simulink model "sm_car_test_ggv_new"  (R2026a)
settings: Solver=ode23t  StopTime=300  MaxStep=0.4  AbsTol=1e-3  EnableMultiTasking=on
PreLoadFcn:
  | % PreLoadFcn Removed for GGV Sweep
PostLoadFcn:
  | % PostLoadFcn Removed for GGV Sweep
InitFcn:
  | sm_car_config_camera;
  | Vehicle = sm_car_vehcfg_checkConfig(Vehicle);
  | sm_car_check_tire_model(bdroot);
StartFcn:
  | tic;
StopFcn:
  | Elapsed_Sim_Time = toc;
  | % disp(['Elapsed Sim Time = ' num2str(Elapsed_Sim_Time)]);
values from neighbouring files (symbols this model uses):
  accel_ramp_rate = 0.1    [sm_car_sweep_ggv_pts.m]
undefined symbols (not defined in the file or in its folder): acc_theta, Axle1D, AxleIn, Camera, Control, drag_frc, Driver, Init, lift_frc, Maneuver, Pedal, Scene, ShaftL1, ShaftL2, ShaftR1, ShaftR2, Visual, X, xy_data_car_side, Y, Z
libraries: sm_lib x270, fl_lib x171, nesl_utility x137, simulink x56, sdl_lib x14, simulink_extras x11, SimscapeFluids_lib x7, Scene_Utilities x6, dspsigops x4, Damper_Element x4, Tire_1x2x x4, ee_lib x3
(part 5 of 20)

== system sm_car_test_ggv_new/World/Scene ==
  CRG Dej : sm_car_scene_crg_dej/CRG Dej  VariantControl=CRG_Dej  geometry=Scene.CRG_Dej.Geometry
  CRG Dej F : sm_car_scene_crg_dej_f/CRG Dej F  VariantControl=CRG_Dej_F  geometry=Scene.CRG_Dej_F.Geometry
  CRG Dej Wide : sm_car_scene_crg_dej_wide/CRG Dej Wide  VariantControl=CRG_Dej_Wide  geometry=Scene.CRG_Dej_Wide.Geometry
  CRG Dej Wide F : sm_car_scene_crg_dej_wide_f/CRG Dej Wide F  VariantControl=CRG_Dej_Wide_F  geometry=Scene.CRG_Dej_Wide_F.Geometry
  CRG Germania : sm_car_scene_crg_germania/CRG Germania  VariantControl=CRG_Germania  geometry=Scene.CRG_Germania.Geometry
  CRG Germania F : sm_car_scene_crg_germania_f/CRG Germania F  VariantControl=CRG_Germania_F  geometry=Scene.CRG_Germania_F.Geometry
  CRG Hockenheim : Subsystem  VariantControl=CRG_Hockenheim  mask{geometry=Scene.CRG_Hockenheim.Geometry}
      mask prompts: geometry "Geometry (structure)"
  CRG Hockenheim F : Subsystem  VariantControl=CRG_Hockenheim_F  mask{geometry=Scene.CRG_Hockenheim_F.Geometry}
      mask prompts: geometry "Geometry (structure)"
  CRG Teste : sm_car_scene_crg_teste/CRG Teste  VariantControl=CRG _Teste  geometry=Scene.CRG_Teste.Geometry
  CRG Teste F : sm_car_scene_crg_teste_f/CRG Teste F  VariantControl=CRG_Teste_F  geometry=Scene.CRG_Teste_F.Geometry
  Double Lane Change : Subsystem  VariantControl=Double_Lane_Change  mask{road=Scene.Double_Lane_Change.Road, dashes=Scene.Double_Lane_Change.Dashes, cones=Scene.Double_Lane_Change.Cones}
      mask prompts: road "Road (structure)"; dashes "Dashes (structure)"; cones "Cones (structure)"
  Double Lane Change ISO3888 : Subsystem  VariantControl=Double_Lane_Change_ISO3888  mask{road=Scene.Double_Lane_Change_ISO3888.Road, dashes=Scene.Double_Lane_Change_ISO3888.Dashes, cones=Scene.Double_Lane_Change_ISO3888.Cones}
      mask prompts: road "Road (structure)"; dashes "Dashes (structure)"; cones "Cones (structure)"
  Plane Grid : Subsystem  VariantControl=Plane_Grid  mask{plane=Scene.Plane_Grid.Plane, grid=Scene.Plane_Grid.Grid}
      mask prompts: plane "Ground Plane (structure)"; grid "Grid (structure)"
  Skidpad : Subsystem  VariantControl=Skidpad  mask{circ_in=Scene.Skidpad.Circle_Inner, circ_out=Scene.Skidpad.Circle_Outer, plane=Scene.Skidpad.Plane}
      mask prompts: circ_in "Circle Inner (structure)"; circ_out "Circle Outer (structure)"; plane "Plane (structure)"
  W : PMIOPort  Side=Left
  Obs : Outport  VectorParamsAs1DForOutWhenUnconnected=off

== system sm_car_test_ggv_new/Camera Frames/Dolly Camera/Off ==
  W : PMIOPort  Side=Left
  R : PMIOPort  Port=2  Side=Right
  connections:
  R/RConn1 -- W/RConn1

== system sm_car_test_ggv_new/Controller/Default/Brake Control ==
  "rBrakePedal " : Inport
  "VehBus " : Inport  Port=2
  Pedal : Subsystem  VariantControl=Pedal
  " Brakes" : Outport  VectorParamsAs1DForOutWhenUnconnected=off

== system sm_car_test_ggv_new/Controller/Default/Driveline Control ==
  Bus Creator : BusCreator  Inputs=1
  Constant : Constant  Value=0
  Driveline : Outport  VectorParamsAs1DForOutWhenUnconnected=off
  wires:
  Bus Creator/1 -> Driveline/1  "Driveline"
  Constant/1 -> Bus Creator/1  "placeholder"

== system sm_car_test_ggv_new/Controller/Default/Power Control ==
  note: For 4 Motor Powertrain only
  note: For 2 Motor Powertrain only
  rAccelPedal : Inport
  VehBus : Inport  Port=2
  StatesEst : Inport  Port=3
  Bus Creator : BusCreator  Inputs=7
  Constant : Constant  Value=trq_ratio_front
  Constant1 : Constant  Value=0
  Constant2 : Constant
  Gain : Gain  Gain=max(Vehicle.Powertrain.Power.Motor.TorqueSpd.trq.Value)
  Gain1 : Gain
  Gain2 : Gain
  Gain3 : Gain  Gain=0.5
  Gain4 : Gain  Gain=0.5
  Product : Product
  Product1 : Product
  Rate Limiter : RateLimiter  RisingSlewLimit=trq_rate_up  FallingSlewLimit=trq_rate_down  SampleTimeMode=inherited
  Terminator : Terminator
  Terminator1 : Terminator
  Power : Outport  VectorParamsAs1DForOutWhenUnconnected=off
  wires:
  Bus Creator/1 -> Power/1  "Power"
  Product1/1 -> Gain2/1, Gain1/1, Bus Creator/4  "MMotorA2Demand"
  Gain/1 -> Rate Limiter/1
  Product/1 -> Gain4/1, Gain3/1, Bus Creator/1  "MMotorA1Demand"
  rAccelPedal/1 -> Gain/1
  VehBus/1 -> Terminator/1
  Constant1/1 -> Bus Creator/7  "MRegenBrakeLimit"
  Rate Limiter/1 -> Product1/1, Product/2
  Constant/1 -> Product/1
  Constant2/1 -> Product1/2
  Gain1/1 -> Bus Creator/5  "MMotorL2Demand"
  Gain2/1 -> Bus Creator/6  "MMotorR2Demand"
  Gain3/1 -> Bus Creator/2  "MMotorL1Demand"
  Gain4/1 -> Bus Creator/3  "MMotorR1Demand"
  StatesEst/1 -> Terminator1/1

== system sm_car_test_ggv_new/Controller/Default/Spring Damper ==
  Bus Creator : BusCreator  Inputs=4
  Bus Creator1 : BusCreator  Inputs=4
  Constant : Constant  Value=[0 0 0 0]
  Constant1 : Constant  Value=[0 0 0 0]
  Demux : Demux
  Demux1 : Demux
  Damper : Outport  VectorParamsAs1DForOutWhenUnconnected=off
  Spring : Outport  Port=2  VectorParamsAs1DForOutWhenUnconnected=off
  wires:
  Constant/1 -> Demux/1
  Demux/3 -> Bus Creator/3  "L2"
  Demux/4 -> Bus Creator/4  "R2"
  Demux/1 -> Bus Creator/1  "L1"
  Demux/2 -> Bus Creator/2  "R1"
  Demux1/2 -> Bus Creator1/2  "R1"
  Demux1/1 -> Bus Creator1/1  "L1"
  Demux1/4 -> Bus Creator1/4  "R2"
  Demux1/3 -> Bus Creator1/3  "L2"
  Constant1/1 -> Demux1/1
  Bus Creator1/1 -> Damper/1  "Damper"
  Bus Creator/1 -> Spring/1  "Spring"

== system sm_car_test_ggv_new/Controller/Default/State Estimation ==
  aSteerWheel : Inport
  VehBus : Inport  Port=2
  Bus Creator : BusCreator  Inputs=6
  Bus Selector : BusSelector  OutputSignals=Chassis.Body.CG.vx,World.vx,World.vy,World.vz,Chassis.Body.CG.aYaw,Chassis.Body.CG.nYaw,Chassis.Body.CG.gx,Chassis.Body.CG.gy,Chassis.SuspA1.LinkageL.Upright.Upright.w,Chassis.SuspA1.LinkageR.Upright.Upright.w,Chassis.SuspA2.LinkageL.Upright.Upright.w,Chassis.SuspA2.LinkageR.Upright.Upright.w
  Compare To Constant : simulink/Logic and Bit Operations/Compare To Constant  relop=>=  const=0.4  OutDataTypeStr=boolean
  Data Type Conversion : DataTypeConversion  OutDataTypeStr=double  SaturateOnIntegerOverflow=off  RndMeth=Floor
  Demux : Demux  Outputs=6
  Rate Transition1 : RateTransition  Deterministic=off  OutPortSampleTime=0.003
  Rate Transition2 : RateTransition  Deterministic=off  OutPortSampleTime=0.003
  Rate Transition3 : RateTransition  Deterministic=off  OutPortSampleTime=0.003
  Sensor Noise Simulation : Subsystem
  Subsystem : Subsystem
  StateEst : Outport
  Out Bus Element : Outport  Port=2  PortName=Meas  Element=Meas
  Out Bus Element1 : Outport  Port=2  PortName=Meas  Element=Input
  Out Bus Element2 : Outport  Port=2  PortName=Meas  Element=State
  wires:
  VehBus/1 -> Bus Selector/1
  Bus Selector/2 -> Sensor Noise Simulation/1(<vx>)  "<vx>"
  Bus Selector/3 -> Sensor Noise Simulation/2(<vy>)  "<vy>"
  Bus Selector/5 -> Sensor Noise Simulation/4(<aYaw>)  "<aYaw>"
  Bus Selector/6 -> Sensor Noise Simulation/5(<nYaw>)  "<nYaw>"
  Bus Selector/7 -> Sensor Noise Simulation/6(<gx>)  "<gx>"
  Bus Selector/8 -> Sensor Noise Simulation/7(<gy>)  "<gy>"
  Bus Selector/9 -> Sensor Noise Simulation/8(<w_fl>)  "<w>"
  Bus Selector/10 -> Sensor Noise Simulation/9(<w_fr>)  "<w>"
  Bus Selector/11 -> Sensor Noise Simulation/10(<w_rl>)  "<w>"
  Bus Selector/12 -> Sensor Noise Simulation/11(<w_rr>)  "<w>"
  aSteerWheel/1 -> Sensor Noise Simulation/12(delta)  "delta"
  Sensor Noise Simulation/2(Meas) -> Out Bus Element/1, Rate Transition2/1  "Measument"
  Sensor Noise Simulation/1(Inputs) -> Out Bus Element1/1, Rate Transition1/1  "Input"
  Bus Selector/4 -> Sensor Noise Simulation/3(<vz>)  "<vz>"
  Data Type Conversion/1 -> Demux/1
  Bus Creator/1 -> Out Bus Element2/1, StateEst/1  "UKF"
  Demux/1 -> Bus Creator/1  "v_x"
  Demux/2 -> Bus Creator/2  "v_y"
  Demux/3 -> Bus Creator/3  "phi"
  Demux/4 -> Bus Creator/4  "phi_dot"
  Demux/5 -> Bus Creator/5  "a_x"
  Demux/6 -> Bus Creator/6  "a_y"
  Compare To Constant/1 -> Rate Transition3/1
  Rate Transition3/1 -> Subsystem/Enable
  Rate Transition1/1 -> Subsystem/1(StateTransitionFcnInputs)
  Rate Transition2/1 -> Subsystem/2(y1)
  Subsystem/1(xhat) -> Data Type Conversion/1
  Bus Selector/1 -> Compare To Constant/1  "<vx>"

== system sm_car_test_ggv_new/Controller/Default/Susp ==
  aSteerWheel : Inport
  vx : Inport  Port=2
  1-D Lookup Table : Lookup_n-D  NumberOfTableDimensions=1  BreakpointsForDimension1=Steer.Gain.vVehicle.Value  Table=Steer.Gain.n.Value  InterpMethod=Linear Lagrange  InternalRulePriority=Speed  RndMeth=Simplest
  Bus Creator{1..4} (4 alike) : BusCreator  Inputs=1
  Gain : Gain  Gain=3.6
  Product : Product
  Saturation : Saturate  UpperLimit=Steer.Limits.aUpper.Value  LowerLimit=Steer.Limits.aLower.Value  LinearizeAsGain=off  ZeroCross=off
  Transfer Fcn (with initial states) : simulink_extras/Additional Linear/Transfer Fcn (with initial states)  N=[1]  D="[1/Steer.fActuatorCutoff.Value  1]"  X0=-1
  SuspA1 : Outport  VectorParamsAs1DForOutWhenUnconnected=off
  SuspA2 : Outport  Port=2  VectorParamsAs1DForOutWhenUnconnected=off
  wires:
  Bus Creator4/1 -> Bus Creator1/1  "Steer"
  Bus Creator2/1 -> Bus Creator3/1  "Steer"
  Bus Creator3/1 -> SuspA2/1  "SuspA2"
  Bus Creator1/1 -> SuspA1/1  "SuspA1"
  aSteerWheel/1 -> Product/1, Bus Creator4/1  "aSteerWheel"
  Saturation/1 -> Bus Creator2/1  "aSteerWheel"
  vx/1 -> Gain/1
  Transfer Fcn (with initial states)/1 -> Product/2
  Product/1 -> Saturation/1
  Gain/1 -> 1-D Lookup Table/1
  1-D Lookup Table/1 -> Transfer Fcn (with initial states)/1

== system sm_car_test_ggv_new/Controller/FeedF_Ctrl/Brake Control ==
  "rBrakePedal " : Inport
  "VehBus " : Inport  Port=2
  Pedal : Subsystem  VariantControl=Pedal
  " Brakes" : Outport  VectorParamsAs1DForOutWhenUnconnected=off

== system sm_car_test_ggv_new/Controller/FeedF_Ctrl/Driveline Control ==
  Bus Creator : BusCreator  Inputs=1
  Constant : Constant  Value=0
  Driveline : Outport  VectorParamsAs1DForOutWhenUnconnected=off
  wires:
  Constant/1 -> Bus Creator/1  "placeholder"
  Bus Creator/1 -> Driveline/1  "Driveline"

== system sm_car_test_ggv_new/Controller/FeedF_Ctrl/Power Control ==
  rAccelPedal : Inport
  VehBus : Inport  Port=2
  aSteerWheel : Inport  Port=3
  Bias : Bias  Bias=512  SaturateOnIntegerOverflow=off
  Bus Creator : BusCreator  Inputs=2
  Bus Selector : BusSelector  OutputSignals=Power.MotorL2.w,Power.MotorR2.w
  Gain : Gain  Gain=max(Control.MotorTrq)
  Gain1 : Gain  Gain=max(Control.MotorTrq)
  Gain3 : Gain  Gain=511/154
  Radians to Degrees : simulink_extras/Transformations/Radians to Degrees
  Subsystem Reference : Subsystem  ReferencedSubsystem=FeedForward  rwheel=Control.WheelRad  L=Control.Wheelbase  StrWhlRatio=Control.StrWheelRatio  Izz=Control.Izz  tr=Control.RearTrack  Gr=Control.GearRatio  MotorT=Control.MotorTrq  MotorW=Control.MotorW  Tf=0.005  Tmax=max(Control.MotorTrq)  Ku=Control.UndersteerGradient
  Power : Outport  VectorParamsAs1DForOutWhenUnconnected=off
  wires:
  Bias/1 -> Subsystem Reference/1
  Gain3/1 -> Bias/1
  Radians to Degrees/1 -> Gain3/1
  Gain1/1 -> Bus Creator/2  "MMotorR2Demand"
  Gain/1 -> Bus Creator/1  "MMotorL2Demand"
  Subsystem Reference/2 -> Gain1/1  "MMotorR2Demand"
  Subsystem Reference/1 -> Gain/1  "MMotorL2Demand"
  Bus Creator/1 -> Power/1
  rAccelPedal/1 -> Subsystem Reference/4  "Throttle[~]"
  aSteerWheel/1 -> Radians to Degrees/1  "Throttle[~]"
  VehBus/1 -> Bus Selector/1
  Bus Selector/1 -> Subsystem Reference/2  "<w>"
  Bus Selector/2 -> Subsystem Reference/3  "<w>"

== system sm_car_test_ggv_new/Controller/FeedF_Ctrl/Spring Damper ==
  Bus Creator : BusCreator  Inputs=4
  Bus Creator1 : BusCreator  Inputs=4
  Constant : Constant  Value=[0 0 0 0]
  Constant1 : Constant  Value=[0 0 0 0]
  Demux : Demux
  Demux1 : Demux
  Damper : Outport  VectorParamsAs1DForOutWhenUnconnected=off
  Spring : Outport  Port=2  VectorParamsAs1DForOutWhenUnconnected=off
  wires:
  Bus Creator/1 -> Spring/1  "Spring"
  Bus Creator1/1 -> Damper/1  "Damper"
  Constant1/1 -> Demux1/1
  Demux1/3 -> Bus Creator1/3  "L2"
  Demux1/4 -> Bus Creator1/4  "R2"
  Demux1/1 -> Bus Creator1/1  "L1"
  Demux1/2 -> Bus Creator1/2  "R1"
  Demux/2 -> Bus Creator/2  "R1"
  Demux/1 -> Bus Creator/1  "L1"
  Demux/4 -> Bus Creator/4  "R2"
  Demux/3 -> Bus Creator/3  "L2"
  Constant/1 -> Demux/1

== system sm_car_test_ggv_new/Controller/FeedF_Ctrl/Susp ==
  aSteerWheel : Inport
  vx : Inport  Port=2
  1-D Lookup Table : Lookup_n-D  NumberOfTableDimensions=1  BreakpointsForDimension1=Steer.Gain.vVehicle.Value  Table=Steer.Gain.n.Value  InterpMethod=Linear Lagrange  InternalRulePriority=Speed  RndMeth=Simplest
  Bus Creator{1..4} (4 alike) : BusCreator  Inputs=1
  Gain : Gain  Gain=3.6
  Product : Product
  Saturation : Saturate  UpperLimit=Steer.Limits.aUpper.Value  LowerLimit=Steer.Limits.aLower.Value  LinearizeAsGain=off  ZeroCross=off
  Transfer Fcn (with initial states) : simulink_extras/Additional Linear/Transfer Fcn (with initial states)  N=[1]  D="[1/Steer.fActuatorCutoff.Value  1]"  X0=-1
  SuspA1 : Outport  VectorParamsAs1DForOutWhenUnconnected=off
  SuspA2 : Outport  Port=2  VectorParamsAs1DForOutWhenUnconnected=off
  wires:
  1-D Lookup Table/1 -> Transfer Fcn (with initial states)/1
  Gain/1 -> 1-D Lookup Table/1
  Product/1 -> Saturation/1
  Transfer Fcn (with initial states)/1 -> Product/2
  vx/1 -> Gain/1
  Saturation/1 -> Bus Creator2/1  "aSteerWheel"
  aSteerWheel/1 -> Bus Creator4/1, Product/1  "aSteerWheel"
  Bus Creator1/1 -> SuspA1/1  "SuspA1"
  Bus Creator3/1 -> SuspA2/1  "SuspA2"
  Bus Creator2/1 -> Bus Creator3/1  "Steer"
  Bus Creator4/1 -> Bus Creator1/1  "Steer"

== system sm_car_test_ggv_new/Controller/NoIMU/Brake Control ==
  "rBrakePedal " : Inport
  "VehBus " : Inport  Port=2
  Pedal : Subsystem  VariantControl=Pedal
  " Brakes" : Outport  VectorParamsAs1DForOutWhenUnconnected=off

== system sm_car_test_ggv_new/Controller/NoIMU/Driveline Control ==
  Bus Creator : BusCreator  Inputs=1
  Constant : Constant  Value=0
  Driveline : Outport  VectorParamsAs1DForOutWhenUnconnected=off
  wires:
  Constant/1 -> Bus Creator/1  "placeholder"
  Bus Creator/1 -> Driveline/1  "Driveline"

== system sm_car_test_ggv_new/Controller/NoIMU/Power Control ==
  rAccelPedal : Inport
  VehBus : Inport  Port=2
  Add1 : Sum
  Bus Creator : BusCreator  Inputs=2
  Bus Creator2 : BusCreator  Inputs=2
  Bus Selector : BusSelector  OutputSignals=Power.Battery.v,Power.MotorL2.i,Power.MotorR2.i
  Constant : Constant
  Current-Torque : Subsystem
  Delay : Delay  DelayLength=1  InputProcessing=Columns as channels (frame based)
  Fuzzy Logic Controller : fuzblock/Fuzzy Logic  Controller  FIS=fis  OutputSampleNumber=101  DataType=double  UseLookupTable=off  NumBreakpoints=10  FuzzifiedInputs=off  RuleFiringStrengths=off  RuleOutputs=off  AggregatedOutputs=off  SimulateUsing=Interpreted execution  OutOfRangeInputValueMessage=warning  NoRuleFiredMessage=warning  EmptyOutputFuzzySetMessage=warning
  Product : Product
  Product1 : Product
  Product2 : Product  Inputs=3
  Saturation : Saturate  UpperLimit=1  LowerLimit=0
  Slip Control : Subsystem  Commented=on
  Subtract : Sum  Inputs=+-
  Sum : Sum  Inputs=|+-
  Tmax : Gain  Gain=1/Tmax/2
  max torque : Constant  Value=Tmax
  Power : Outport  VectorParamsAs1DForOutWhenUnconnected=off
  wires:
  VehBus/1 -> Slip Control/1(VehBus), Bus Selector/1
  Bus Creator/1 -> Power/1  "Power"
  rAccelPedal/1 -> Sum/1, Product2/1  "Throttle[~]"
  Bus Selector/1 -> Current-Torque/1(V)  "<v>"
  Bus Selector/2 -> Current-Torque/2(Il)  "<i>"
  Bus Selector/3 -> Current-Torque/3(Ir)  "<i>"
  Fuzzy Logic Controller/1 -> Add1/2
  Current-Torque/1(Out1) -> Tmax/1  "Treal[Nm]"
  Bus Creator2/1 -> ?
  Product2/1 -> Product/1, Product1/1  "MDemand[Nm]"
  Tmax/1 -> Saturation/1
  Saturation/1 -> Sum/2  "Treal[%]"
  max torque/1 -> Product2/3
  Add1/1 -> Product2/2
  Sum/1 -> Delay/1, Subtract/1, Bus Creator2/1
  Delay/1 -> Subtract/2
  Subtract/1 -> Bus Creator2/2
  Constant/1 -> Add1/1
  Product/1 -> Bus Creator/2  "MMotorR2Demand"
  Product1/1 -> Bus Creator/1  "MMotorL2Demand"
  Slip Control/1(Out1) -> Product1/2
  Slip Control/2(Out2) -> Product/2

== system sm_car_test_ggv_new/Controller/NoIMU/Spring Damper ==
  Bus Creator : BusCreator  Inputs=4
  Bus Creator1 : BusCreator  Inputs=4
  Constant : Constant  Value=[0 0 0 0]
  Constant1 : Constant  Value=[0 0 0 0]
  Demux : Demux
  Demux1 : Demux
  Damper : Outport  VectorParamsAs1DForOutWhenUnconnected=off
  Spring : Outport  Port=2  VectorParamsAs1DForOutWhenUnconnected=off
  wires:
  Bus Creator/1 -> Spring/1  "Spring"
  Bus Creator1/1 -> Damper/1  "Damper"
  Constant1/1 -> Demux1/1
  Demux1/3 -> Bus Creator1/3  "L2"
  Demux1/4 -> Bus Creator1/4  "R2"
  Demux1/1 -> Bus Creator1/1  "L1"
  Demux1/2 -> Bus Creator1/2  "R1"
  Demux/2 -> Bus Creator/2  "R1"
  Demux/1 -> Bus Creator/1  "L1"
  Demux/4 -> Bus Creator/4  "R2"
  Demux/3 -> Bus Creator/3  "L2"
  Constant/1 -> Demux/1

== system sm_car_test_ggv_new/Controller/NoIMU/Susp ==
  aSteerWheel : Inport
  vx : Inport  Port=2
  1-D Lookup Table : Lookup_n-D  NumberOfTableDimensions=1  BreakpointsForDimension1=Steer.Gain.vVehicle.Value  Table=Steer.Gain.n.Value  InterpMethod=Linear Lagrange  InternalRulePriority=Speed  RndMeth=Simplest
  Bus Creator{1..4} (4 alike) : BusCreator  Inputs=1
  Gain : Gain  Gain=3.6
  Product : Product
  Saturation : Saturate  UpperLimit=Steer.Limits.aUpper.Value  LowerLimit=Steer.Limits.aLower.Value  LinearizeAsGain=off  ZeroCross=off
  Transfer Fcn (with initial states) : simulink_extras/Additional Linear/Transfer Fcn (with initial states)  N=[1]  D="[1/Steer.fActuatorCutoff.Value  1]"  X0=-1
  SuspA1 : Outport  VectorParamsAs1DForOutWhenUnconnected=off
  SuspA2 : Outport  Port=2  VectorParamsAs1DForOutWhenUnconnected=off
  wires:
  1-D Lookup Table/1 -> Transfer Fcn (with initial states)/1
  Gain/1 -> 1-D Lookup Table/1
  Product/1 -> Saturation/1
  Transfer Fcn (with initial states)/1 -> Product/2
  vx/1 -> Gain/1
  Saturation/1 -> Bus Creator2/1  "aSteerWheel"
  aSteerWheel/1 -> Bus Creator4/1, Product/1  "aSteerWheel"
  Bus Creator1/1 -> SuspA1/1  "SuspA1"
  Bus Creator3/1 -> SuspA2/1  "SuspA2"
  Bus Creator2/1 -> Bus Creator3/1  "Steer"
  Bus Creator4/1 -> Bus Creator1/1  "Steer"

== system sm_car_test_ggv_new/Controller/Slip_Ctrl/Brake Control ==
  "rBrakePedal " : Inport
  "VehBus " : Inport  Port=2
  Pedal : Subsystem  VariantControl=Pedal
  " Brakes" : Outport  VectorParamsAs1DForOutWhenUnconnected=off

== system sm_car_test_ggv_new/Controller/Slip_Ctrl/Driveline Control ==
  Bus Creator : BusCreator  Inputs=1
  Constant : Constant  Value=0
  Driveline : Outport  VectorParamsAs1DForOutWhenUnconnected=off
  wires:
  Constant/1 -> Bus Creator/1  "placeholder"
  Bus Creator/1 -> Driveline/1  "Driveline"

== system sm_car_test_ggv_new/Controller/Slip_Ctrl/Power Control ==
  rAccelPedal : Inport
  VehBus : Inport  Port=2
  Bus Creator : BusCreator  Inputs=2
  Bus Selector : BusSelector  OutputSignals=Chassis.Body.CG.vx,Chassis.SuspA2.LinkageL.Upright.Upright.w,Chassis.SuspA2.LinkageR.Upright.Upright.w,Chassis.Body.CG.gx,Chassis.Body.CG.gy,Chassis.Body.CG.nYaw
  Gain : Gain  Gain=max(Control.MotorTrq)
  Gain1 : Gain  Gain=max(Control.MotorTrq)
  Slip Control : Subsystem  TreatAsAtomicUnit=on  ReferencedSubsystem=Slip_Control  Gr=Control.GearRatio  MotorT=Control.MotorTrq  MotorW=Control.MotorW  rwheel=Control.WheelRad  tr=Control.RearTrack  a=Control.FrontTrackToCG  a_cop=Control.FrontTrackToCoP  Af=Control.FrontalArea  P=800  I=6000  N=100  D=11  vx_th=Control.ActivationVelocity  cd=Control.LiftCoef  g=Control.GravitationAcc  h_CG=Control.CGHeight  L=Control.Wheelbase  m=Control.Mass  ro=Control.AirDensity  Tmax=max(Control.MotorTrq)  Load_Ref=Control.LoadRef  Slip_Ref=0.1*ones(18,1)
  Power : Outport  VectorParamsAs1DForOutWhenUnconnected=off
  wires:
  Slip Control/2 -> Gain1/1  "MMotorR2Demand"
  Slip Control/1 -> Gain/1  "MMotorL2Demand"
  Bus Creator/1 -> Power/1
  Bus Selector/6 -> Slip Control/6  "<nYaw>"
  Bus Selector/4 -> Slip Control/4  "<gx>"
  Bus Selector/5 -> Slip Control/5  "<gy>"
  Bus Selector/3 -> Slip Control/3  "<w>"
  Bus Selector/1 -> Slip Control/1  "<vx>"
  rAccelPedal/1 -> Slip Control/7  "Throttle[~]"
  VehBus/1 -> Bus Selector/1
  Bus Selector/2 -> Slip Control/2  "<w>"
  Gain/1 -> Bus Creator/1  "MMotorL2Demand"
  Gain1/1 -> Bus Creator/2  "MMotorR2Demand"

== system sm_car_test_ggv_new/Controller/Slip_Ctrl/Spring Damper ==
  Bus Creator : BusCreator  Inputs=4
  Bus Creator1 : BusCreator  Inputs=4
  Constant : Constant  Value=[0 0 0 0]
  Constant1 : Constant  Value=[0 0 0 0]
  Demux : Demux
  Demux1 : Demux
  Damper : Outport  VectorParamsAs1DForOutWhenUnconnected=off
  Spring : Outport  Port=2  VectorParamsAs1DForOutWhenUnconnected=off
  wires:
  Bus Creator/1 -> Spring/1  "Spring"
  Bus Creator1/1 -> Damper/1  "Damper"
  Constant1/1 -> Demux1/1
  Demux1/3 -> Bus Creator1/3  "L2"
  Demux1/4 -> Bus Creator1/4  "R2"
  Demux1/1 -> Bus Creator1/1  "L1"
  Demux1/2 -> Bus Creator1/2  "R1"
  Demux/2 -> Bus Creator/2  "R1"
  Demux/1 -> Bus Creator/1  "L1"
  Demux/4 -> Bus Creator/4  "R2"
  Demux/3 -> Bus Creator/3  "L2"
  Constant/1 -> Demux/1

== system sm_car_test_ggv_new/Controller/Slip_Ctrl/Susp ==
  aSteerWheel : Inport
  vx : Inport  Port=2
  1-D Lookup Table : Lookup_n-D  NumberOfTableDimensions=1  BreakpointsForDimension1=Steer.Gain.vVehicle.Value  Table=Steer.Gain.n.Value  InterpMethod=Linear Lagrange  InternalRulePriority=Speed  RndMeth=Simplest
  Bus Creator{1..4} (4 alike) : BusCreator  Inputs=1
  Gain : Gain  Gain=3.6
  Product : Product
  Saturation : Saturate  UpperLimit=Steer.Limits.aUpper.Value  LowerLimit=Steer.Limits.aLower.Value  LinearizeAsGain=off  ZeroCross=off
  Transfer Fcn (with initial states) : simulink_extras/Additional Linear/Transfer Fcn (with initial states)  N=[1]  D="[1/Steer.fActuatorCutoff.Value  1]"  X0=-1
  SuspA1 : Outport  VectorParamsAs1DForOutWhenUnconnected=off
  SuspA2 : Outport  Port=2  VectorParamsAs1DForOutWhenUnconnected=off
  wires:
  1-D Lookup Table/1 -> Transfer Fcn (with initial states)/1
  Gain/1 -> 1-D Lookup Table/1
  Product/1 -> Saturation/1
  Transfer Fcn (with initial states)/1 -> Product/2
  vx/1 -> Gain/1
  Saturation/1 -> Bus Creator2/1  "aSteerWheel"
  aSteerWheel/1 -> Bus Creator4/1, Product/1  "aSteerWheel"
  Bus Creator1/1 -> SuspA1/1  "SuspA1"
  Bus Creator3/1 -> SuspA2/1  "SuspA2"
  Bus Creator2/1 -> Bus Creator3/1  "Steer"
  Bus Creator4/1 -> Bus Creator1/1  "Steer"

== system sm_car_test_ggv_new/Controller/Slip_Ctrl_V2/Brake Control ==
  "rBrakePedal " : Inport
  "VehBus " : Inport  Port=2
  Pedal : Subsystem  VariantControl=Pedal
  " Brakes" : Outport  VectorParamsAs1DForOutWhenUnconnected=off

== system sm_car_test_ggv_new/Controller/Slip_Ctrl_V2/Driveline Control ==
  Bus Creator : BusCreator  Inputs=1
  Constant : Constant  Value=0
  Driveline : Outport  VectorParamsAs1DForOutWhenUnconnected=off
  wires:
  Bus Creator/1 -> Driveline/1  "Driveline"
  Constant/1 -> Bus Creator/1  "placeholder"

== system sm_car_test_ggv_new/Controller/Slip_Ctrl_V2/Power Control ==
  rAccelPedal : Inport
  VehBus : Inport  Port=2
  Bus Creator : BusCreator  Inputs=2
  Bus Selector : BusSelector  OutputSignals=Chassis.Body.CG.vx,Chassis.SuspA2.LinkageL.Upright.Upright.w,Chassis.SuspA2.LinkageR.Upright.Upright.w,Chassis.Body.CG.gx,Chassis.Body.CG.gy,Chassis.Body.CG.nYaw
  Gain : Gain  Gain=max(Control.MotorTrq)
  Gain1 : Gain  Gain=max(Control.MotorTrq)
  Slip Control : Subsystem  TreatAsAtomicUnit=on  ReferencedSubsystem=Slip_Control  Gr=Control.GearRatio  MotorT=Control.MotorTrq  MotorW=Control.MotorW  rwheel=Control.WheelRad  tr=Control.RearTrack  a=Control.FrontTrackToCG  a_cop=Control.FrontTrackToCoP  Af=Control.FrontalArea  P=800  I=6000  N=100  D=11  vx_th=Control.ActivationVelocity  cd=Control.LiftCoef  g=Control.GravitationAcc  h_CG=Control.CGHeight  L=Control.Wheelbase  m=Control.Mass  ro=Control.AirDensity  Tmax=max(Control.MotorTrq)  Load_Ref=Control.LoadRef  Slip_Ref=Control.SlipRef
  Power : Outport  VectorParamsAs1DForOutWhenUnconnected=off
  wires:
  VehBus/1 -> Bus Selector/1
  Bus Creator/1 -> Power/1
  Gain/1 -> Bus Creator/1  "MMotorL2Demand"
  Gain1/1 -> Bus Creator/2  "MMotorR2Demand"
  Bus Selector/1 -> Slip Control/1  "<vx>"
  Bus Selector/2 -> Slip Control/2  "<w>"
  Bus Selector/3 -> Slip Control/3  "<w>"
  rAccelPedal/1 -> Slip Control/7  "Throttle[~]"
  Slip Control/1 -> Gain/1  "MMotorL2Demand"
  Slip Control/2 -> Gain1/1  "MMotorR2Demand"
  Bus Selector/4 -> Slip Control/4  "<gx>"
  Bus Selector/5 -> Slip Control/5  "<gy>"
  Bus Selector/6 -> Slip Control/6  "<nYaw>"

== system sm_car_test_ggv_new/Controller/Slip_Ctrl_V2/Spring Damper ==
  Bus Creator : BusCreator  Inputs=4
  Bus Creator1 : BusCreator  Inputs=4
  Constant : Constant  Value=[0 0 0 0]
  Constant1 : Constant  Value=[0 0 0 0]
  Demux : Demux
  Demux1 : Demux
  Damper : Outport  VectorParamsAs1DForOutWhenUnconnected=off
  Spring : Outport  Port=2  VectorParamsAs1DForOutWhenUnconnected=off
  wires:
  Constant/1 -> Demux/1
  Demux/3 -> Bus Creator/3  "L2"
  Demux/4 -> Bus Creator/4  "R2"
  Demux/1 -> Bus Creator/1  "L1"
  Demux/2 -> Bus Creator/2  "R1"
  Demux1/2 -> Bus Creator1/2  "R1"
  Demux1/1 -> Bus Creator1/1  "L1"
  Demux1/4 -> Bus Creator1/4  "R2"
  Demux1/3 -> Bus Creator1/3  "L2"
  Constant1/1 -> Demux1/1
  Bus Creator1/1 -> Damper/1  "Damper"
  Bus Creator/1 -> Spring/1  "Spring"

== system sm_car_test_ggv_new/Controller/Slip_Ctrl_V2/Susp ==
  aSteerWheel : Inport
  vx : Inport  Port=2
  1-D Lookup Table : Lookup_n-D  NumberOfTableDimensions=1  BreakpointsForDimension1=Steer.Gain.vVehicle.Value  Table=Steer.Gain.n.Value  InterpMethod=Linear Lagrange  InternalRulePriority=Speed  RndMeth=Simplest
  Bus Creator{1..4} (4 alike) : BusCreator  Inputs=1
  Gain : Gain  Gain=3.6
  Product : Product
  Saturation : Saturate  UpperLimit=Steer.Limits.aUpper.Value  LowerLimit=Steer.Limits.aLower.Value  LinearizeAsGain=off  ZeroCross=off
  Transfer Fcn (with initial states) : simulink_extras/Additional Linear/Transfer Fcn (with initial states)  N=[1]  D="[1/Steer.fActuatorCutoff.Value  1]"  X0=-1
  SuspA1 : Outport  VectorParamsAs1DForOutWhenUnconnected=off
  SuspA2 : Outport  Port=2  VectorParamsAs1DForOutWhenUnconnected=off
  wires:
  Bus Creator4/1 -> Bus Creator1/1  "Steer"
  Bus Creator2/1 -> Bus Creator3/1  "Steer"
  Bus Creator3/1 -> SuspA2/1  "SuspA2"
  Bus Creator1/1 -> SuspA1/1  "SuspA1"
  aSteerWheel/1 -> Product/1, Bus Creator4/1  "aSteerWheel"
  Saturation/1 -> Bus Creator2/1  "aSteerWheel"
  vx/1 -> Gain/1
  Transfer Fcn (with initial states)/1 -> Product/2
  Product/1 -> Saturation/1
  Gain/1 -> 1-D Lookup Table/1
  1-D Lookup Table/1 -> Transfer Fcn (with initial states)/1

== system sm_car_test_ggv_new/Controller/TrqVec 4Motor/Brake Control ==
  "rBrakePedal " : Inport
  "VehBus " : Inport  Port=2
  ABS : Subsystem  VariantControl=ABS  mask{abs_tire_radiusF=abs_tire_radiusF, abs_tire_radiusR=abs_tire_radiusR}
      mask prompts: abs_tire_radiusF "Tire Radius Front (m)"; abs_tire_radiusR "Tire Radius Rear (m)"
  Pedal : Subsystem  VariantControl=Pedal
  Pressure : Subsystem  VariantControl=Pressure
  " Brakes" : Outport  VectorParamsAs1DForOutWhenUnconnected=off

== system sm_car_test_ggv_new/Controller/TrqVec 4Motor/Driveline Control ==
  Bus Creator : BusCreator  Inputs=1
  Constant : Constant  Value=0
  Driveline : Outport  VectorParamsAs1DForOutWhenUnconnected=off
  wires:
  Bus Creator/1 -> Driveline/1  "Driveline"
  Constant/1 -> Bus Creator/1  "placeholder"

== system sm_car_test_ggv_new/Controller/TrqVec 4Motor/Power_TqVec ==
  In Bus Element6 : Inport  PortName=DrvBus  Element=rAccelPedal
  In Bus Element2 : Inport  PortName=DrvBus  Element=aSteerWheel
  In Bus Element3 : Inport  PortName=DrvBus  Element=rBrakePedal
  In Bus Element : Inport  Port=2  PortName=VehBus  Element=Chassis.Body.CG.vx
  In Bus Element1 : Inport  Port=2  PortName=VehBus  Element=Power.MotorL2.w
  In Bus Element8 : Inport  Port=2  PortName=VehBus  Element=Power.MotorR2.w
  In Bus Element5 : Inport  Port=2  PortName=VehBus  Element=World.nYaw
  Bus Creator : BusCreator  Inputs=5
  Constant : Constant  Value=Control.trq_ratio_front
  Constant2 : Constant  Value=1-Control.trq_ratio_front
  Gain1 : Gain  Gain=1600
  Gain3 : Gain  Gain=0.5
  Gain4 : Gain  Gain=0.5
  Product : Product
  Product1 : Product
  Rate Limiter : RateLimiter  RisingSlewLimit=300  FallingSlewLimit=-5000  SampleTimeMode=inherited
  Torque Vectoring : Subsystem  mask(Torque Vectoring, Rear Wheels){vx_enable=Control.vx_enable, aSteerWheel_enable=Control.aSteerWheel_enable, aStr_to_aWhl=Control.aStr_to_aWhl, max_torque_delta=Control.max_torque_delta, P=Control.pGain, I=Control.iGain}
      mask prompts: vx_enable "Speed to enable (m/s)"; aSteerWheel_enable "Steering wheel angle to enable (rad)"; aStr_to_aWhl "Steering Ratio (Wheel/Steering Wheel)"; max_torque_delta "Max Torque Split (N*m)"; P "Simulink:masks:ProportionalP_MP"; I "Simulink:masks:IntegralI_MP"
      mask help: Basic torque vectoring algorithm which applies opposing offsets to the commanded torque of the rear wheels based on the error between the vehicle slip angle and the angle of the steered wheels.
      mask TypeOptions vx_enable: Enable/Enable vx/const
      mask TypeOptions aSteerWheel_enable: Enable/const/Value
      mask TypeOptions aStr_to_aWhl:
      | Vehicle Slip Angle Error/Steering Wheel
      | to Driving Wheel/Gain
      mask TypeOptions max_torque_delta: Max Delta Torque/Value
      mask TypeOptions P: PID Controller/P
      mask TypeOptions I: PID Controller/I
      mask DialogControl P Prompt: Proportional (P):
      mask DialogControl I Prompt: Integral (I):
  Power : Outport  VectorParamsAs1DForOutWhenUnconnected=off
  wires:
  Torque Vectoring/2(trqR2) -> Bus Creator/5  "MMotorR2Demand"
  Torque Vectoring/1(trqL2) -> Bus Creator/4  "MMotorL2Demand"
  In Bus Element3/1 -> Torque Vectoring/7(rBrake)
  In Bus Element5/1 -> Torque Vectoring/6(nYaw)
  In Bus Element8/1 -> Torque Vectoring/5(wR2)
  In Bus Element1/1 -> Torque Vectoring/4(wL2)
  In Bus Element2/1 -> Torque Vectoring/3(aSteerWheel)
  In Bus Element/1 -> Torque Vectoring/2(vx)
  Product1/1 -> Torque Vectoring/1(trqA2)
  Bus Creator/1 -> Power/1  "Power"
  Gain4/1 -> Bus Creator/3  "MMotorR1Demand"
  Gain3/1 -> Bus Creator/2  "MMotorL1Demand"
  Product/1 -> Gain4/1, Gain3/1, Bus Creator/1  "MMotorA1Demand"
  Constant2/1 -> Product1/2
  Constant/1 -> Product/1
  Rate Limiter/1 -> Product/2, Product1/1
  In Bus Element6/1 -> Gain1/1
  Gain1/1 -> Rate Limiter/1

== system sm_car_test_ggv_new/Controller/TrqVec 4Motor/Spring Damper ==
  Bus Creator : BusCreator  Inputs=4
  Bus Creator1 : BusCreator  Inputs=4
  Constant : Constant  Value=[0 0 0 0]
  Constant1 : Constant  Value=[0 0 0 0]
  Demux : Demux
  Demux1 : Demux
  Damper : Outport  VectorParamsAs1DForOutWhenUnconnected=off
  Spring : Outport  Port=2  VectorParamsAs1DForOutWhenUnconnected=off
  wires:
  Constant/1 -> Demux/1
  Demux/3 -> Bus Creator/3  "L2"
  Demux/4 -> Bus Creator/4  "R2"
  Demux/1 -> Bus Creator/1  "L1"
  Demux/2 -> Bus Creator/2  "R1"
  Demux1/2 -> Bus Creator1/2  "R1"
  Demux1/1 -> Bus Creator1/1  "L1"
  Demux1/4 -> Bus Creator1/4  "R2"
  Demux1/3 -> Bus Creator1/3  "L2"
  Constant1/1 -> Demux1/1
  Bus Creator1/1 -> Damper/1  "Damper"
  Bus Creator/1 -> Spring/1  "Spring"

== system sm_car_test_ggv_new/Controller/TrqVec 4Motor/Susp ==
  aSteerWheel : Inport
  vx : Inport  Port=2
  1-D Lookup Table : Lookup_n-D  NumberOfTableDimensions=1  BreakpointsForDimension1=Steer.Gain.vVehicle.Value  Table=Steer.Gain.n.Value  InterpMethod=Linear Lagrange  InternalRulePriority=Speed  RndMeth=Simplest
  Bus Creator{1..4} (4 alike) : BusCreator  Inputs=1
  Gain : Gain  Gain=3.6
  Product : Product
  Saturation : Saturate  UpperLimit=Steer.Limits.aUpper.Value  LowerLimit=Steer.Limits.aLower.Value  LinearizeAsGain=off  ZeroCross=off
  Transfer Fcn (with initial states) : simulink_extras/Additional Linear/Transfer Fcn (with initial states)  N=[1]  D="[1/Steer.fActuatorCutoff.Value  1]"  X0=-1
  SuspA1 : Outport  VectorParamsAs1DForOutWhenUnconnected=off
  SuspA2 : Outport  Port=2  VectorParamsAs1DForOutWhenUnconnected=off
  wires:
  Bus Creator4/1 -> Bus Creator1/1  "Steer"
  Bus Creator2/1 -> Bus Creator3/1  "Steer"
  Bus Creator3/1 -> SuspA2/1  "SuspA2"
  Bus Creator1/1 -> SuspA1/1  "SuspA1"
  aSteerWheel/1 -> Product/1, Bus Creator4/1  "aSteerWheel"
  Saturation/1 -> Bus Creator2/1  "aSteerWheel"
  vx/1 -> Gain/1
  Transfer Fcn (with initial states)/1 -> Product/2
  Product/1 -> Saturation/1
  Gain/1 -> 1-D Lookup Table/1
  1-D Lookup Table/1 -> Transfer Fcn (with initial states)/1

== system sm_car_test_ggv_new/Controller/TrqVec_FLC/Brake Control ==
  "rBrakePedal " : Inport
  "VehBus " : Inport  Port=2
  Pedal : Subsystem  VariantControl=Pedal
  " Brakes" : Outport  VectorParamsAs1DForOutWhenUnconnected=off

== system sm_car_test_ggv_new/Controller/TrqVec_FLC/Driveline Control ==
  Bus Creator : BusCreator  Inputs=1
  Constant : Constant  Value=0
  Driveline : Outport  VectorParamsAs1DForOutWhenUnconnected=off
  wires:
  Bus Creator/1 -> Driveline/1  "Driveline"
  Constant/1 -> Bus Creator/1  "placeholder"

== system sm_car_test_ggv_new/Controller/TrqVec_FLC/Power Control ==
  rAccelPedal : Inport
  VehBus : Inport  Port=2
  aSteerWheel : Inport  Port=3
  Bus Creator : BusCreator  Inputs=2
  Bus Selector : BusSelector  OutputSignals=Chassis.Body.CG.vx,Chassis.Body.CG.gy,Chassis.Body.CG.nYaw,Power.MotorL2.w,Power.MotorR2.w
  Gain : Gain  Gain=max(Control.MotorTrq)
  Gain1 : Gain  Gain=max(Control.MotorTrq)
  Gain2 : Gain  Gain=1/9.80665
  TV_FLC : Subsystem  TreatAsAtomicUnit=on  ReferencedSubsystem=TV_FLC  StrWheelRatio=Control.StrWheelRatio  Ku=Control.UndersteerGradient  L=Control.Wheelbase  rwheel=Control.WheelRad  Gr=Control.GearRatio  fis=Control.FuzzySystem  Kp=250  tr=Control.RearTrack  alpha_max=Control.SlipTh  MotorT=Control.MotorTrq  MotorW=Control.MotorW  F=Control.F  Tmax=max(Control.MotorTrq)
  Power : Outport  VectorParamsAs1DForOutWhenUnconnected=off
  wires:
  VehBus/1 -> Bus Selector/1
  Bus Selector/1 -> TV_FLC/2  "<vx>"
  Bus Selector/2 -> Gain2/1  "<gy>"
  Bus Selector/3 -> TV_FLC/4  "<nYaw>"
  Bus Selector/4 -> TV_FLC/5  "<w>"
  Bus Selector/5 -> TV_FLC/6  "<w>"
  rAccelPedal/1 -> TV_FLC/7  "Throttle[~]"
  Bus Creator/1 -> Power/1
  TV_FLC/1 -> Gain/1  "MMotorL2Demand"
  TV_FLC/2 -> Gain1/1  "MMotorR2Demand"
  Gain/1 -> Bus Creator/1  "MMotorL2Demand"
  Gain1/1 -> Bus Creator/2  "MMotorR2Demand"
  Gain2/1 -> TV_FLC/3
  aSteerWheel/1 -> TV_FLC/1

== system sm_car_test_ggv_new/Controller/TrqVec_FLC/Spring Damper ==
  Bus Creator : BusCreator  Inputs=4
  Bus Creator1 : BusCreator  Inputs=4
  Constant : Constant  Value=[0 0 0 0]
  Constant1 : Constant  Value=[0 0 0 0]
  Demux : Demux
  Demux1 : Demux
  Damper : Outport  VectorParamsAs1DForOutWhenUnconnected=off
  Spring : Outport  Port=2  VectorParamsAs1DForOutWhenUnconnected=off
  wires:
  Constant/1 -> Demux/1
  Demux/3 -> Bus Creator/3  "L2"
  Demux/4 -> Bus Creator/4  "R2"
  Demux/1 -> Bus Creator/1  "L1"
  Demux/2 -> Bus Creator/2  "R1"
  Demux1/2 -> Bus Creator1/2  "R1"
  Demux1/1 -> Bus Creator1/1  "L1"
  Demux1/4 -> Bus Creator1/4  "R2"
  Demux1/3 -> Bus Creator1/3  "L2"
  Constant1/1 -> Demux1/1
  Bus Creator1/1 -> Damper/1  "Damper"
  Bus Creator/1 -> Spring/1  "Spring"

== system sm_car_test_ggv_new/Controller/TrqVec_FLC/Susp ==
  aSteerWheel : Inport
  vx : Inport  Port=2
  1-D Lookup Table : Lookup_n-D  NumberOfTableDimensions=1  BreakpointsForDimension1=Steer.Gain.vVehicle.Value  Table=Steer.Gain.n.Value  InterpMethod=Linear Lagrange  InternalRulePriority=Speed  RndMeth=Simplest
  Bus Creator{1..4} (4 alike) : BusCreator  Inputs=1
  Gain : Gain  Gain=3.6
  Product : Product
  Saturation : Saturate  UpperLimit=Steer.Limits.aUpper.Value  LowerLimit=Steer.Limits.aLower.Value  LinearizeAsGain=off  ZeroCross=off
  Transfer Fcn (with initial states) : simulink_extras/Additional Linear/Transfer Fcn (with initial states)  N=[1]  D="[1/Steer.fActuatorCutoff.Value  1]"  X0=-1
  SuspA1 : Outport  VectorParamsAs1DForOutWhenUnconnected=off
  SuspA2 : Outport  Port=2  VectorParamsAs1DForOutWhenUnconnected=off
  wires:
  Bus Creator4/1 -> Bus Creator1/1  "Steer"
  Bus Creator2/1 -> Bus Creator3/1  "Steer"
  Bus Creator3/1 -> SuspA2/1  "SuspA2"
  Bus Creator1/1 -> SuspA1/1  "SuspA1"
  aSteerWheel/1 -> Product/1, Bus Creator4/1  "aSteerWheel"
  Saturation/1 -> Bus Creator2/1  "aSteerWheel"
  vx/1 -> Gain/1
  Transfer Fcn (with initial states)/1 -> Product/2
  Product/1 -> Saturation/1
  Gain/1 -> 1-D Lookup Table/1
  1-D Lookup Table/1 -> Transfer Fcn (with initial states)/1

== system sm_car_test_ggv_new/Controller/TrqVec_FLC_V2/Brake Control ==
  "rBrakePedal " : Inport
  "VehBus " : Inport  Port=2
  Pedal : Subsystem  VariantControl=Pedal
  " Brakes" : Outport  VectorParamsAs1DForOutWhenUnconnected=off

== system sm_car_test_ggv_new/Controller/TrqVec_FLC_V2/Driveline Control ==
  Bus Creator : BusCreator  Inputs=1
  Constant : Constant  Value=0
  Driveline : Outport  VectorParamsAs1DForOutWhenUnconnected=off
  wires:
  Constant/1 -> Bus Creator/1  "placeholder"
  Bus Creator/1 -> Driveline/1  "Driveline"

== system sm_car_test_ggv_new/Controller/TrqVec_FLC_V2/Power Control ==
  rAccelPedal : Inport
  VehBus : Inport  Port=2
  aSteerWheel : Inport  Port=3
  Bus Creator : BusCreator  Inputs=2
  Bus Selector : BusSelector  OutputSignals=Chassis.Body.CG.vx,Chassis.Body.CG.gx,Chassis.Body.CG.gy,Chassis.Body.CG.nYaw,Chassis.SuspA2.LinkageL.Upright.Upright.w,Chassis.SuspA2.LinkageR.Upright.Upright.w,Chassis.Body.CG.vy
  Controler type : Constant  Value=2
  Gain : Gain  Gain=max(Control.MotorTrq)
  Gain1 : Gain  Gain=max(Control.MotorTrq)
  Gain2 : Gain  Gain=1/9.80665
  TV FLC V2 : Subsystem  TreatAsAtomicUnit=on  ReferencedSubsystem=TV_FLC_V2  MotorT=Control.MotorTrq  Gr=Control.GearRatio  MotorW=Control.MotorW  rwheel=Control.WheelRad  tr=Control.RearTrack  a=Control.FrontTrackToCG  a_cop=Control.FrontTrackToCoP  Af=Control.FrontalArea  cd=Control.LiftCoef  g=Control.GravitationalAcc  ro=Control.AirDensity  m=Control.Mass  h_CG=Control.CGHeight  L=Control.Wheelbase  Gain=Control.StrWheelRatio  Ku=Control.UndersteerGradient  F=Control.F  P=Control.Proportional_P  I=Control.Integral_I  D=Control.Derivative_D  N=Control.Filter_N  Load_Ref=Control.LoadRef  Slip_Ref=Control.SlipRef  FIS_1=Control.FuzzySystem_1  FIS_2=Control.FuzzySystem_2  FIS_3=Control.FuzzySystem_3  vx_th=Control.ActivationVelocity  Tmax=max(Control.MotorTrq)  C_alpha_F=Control.CalphaF
  Power : Outport  VectorParamsAs1DForOutWhenUnconnected=off
  wires:
  aSteerWheel/1 -> TV FLC V2/1
  Gain2/1 -> TV FLC V2/4
  Gain1/1 -> Bus Creator/2  "MMotorR2Demand"
  Gain/1 -> Bus Creator/1  "MMotorL2Demand"
  TV FLC V2/2 -> Gain1/1  "MMotorR2Demand"
  TV FLC V2/1 -> Gain/1  "MMotorL2Demand"
  Bus Creator/1 -> Power/1
  rAccelPedal/1 -> TV FLC V2/9  "Throttle[~]"
  Bus Selector/6 -> TV FLC V2/7  "<w>"
  Bus Selector/5 -> TV FLC V2/6  "<w>"
  Bus Selector/4 -> TV FLC V2/5  "<nYaw>"
  Bus Selector/3 -> Gain2/1  "<gy>"
  Bus Selector/1 -> TV FLC V2/2  "<vx>"
  VehBus/1 -> Bus Selector/1
  Bus Selector/2 -> TV FLC V2/3  "<gx>"
  Bus Selector/7 -> TV FLC V2/8  "<vy>"
  Controler type/1 -> TV FLC V2/10

== system sm_car_test_ggv_new/Controller/TrqVec_FLC_V2/Spring Damper ==
  Bus Creator : BusCreator  Inputs=4
  Bus Creator1 : BusCreator  Inputs=4
  Constant : Constant  Value=[0 0 0 0]
  Constant1 : Constant  Value=[0 0 0 0]
  Demux : Demux
  Demux1 : Demux
  Damper : Outport  VectorParamsAs1DForOutWhenUnconnected=off
  Spring : Outport  Port=2  VectorParamsAs1DForOutWhenUnconnected=off
  wires:
  Bus Creator/1 -> Spring/1  "Spring"
  Bus Creator1/1 -> Damper/1  "Damper"
  Constant1/1 -> Demux1/1
  Demux1/3 -> Bus Creator1/3  "L2"
  Demux1/4 -> Bus Creator1/4  "R2"
  Demux1/1 -> Bus Creator1/1  "L1"
  Demux1/2 -> Bus Creator1/2  "R1"
  Demux/2 -> Bus Creator/2  "R1"
  Demux/1 -> Bus Creator/1  "L1"
  Demux/4 -> Bus Creator/4  "R2"
  Demux/3 -> Bus Creator/3  "L2"
  Constant/1 -> Demux/1

== system sm_car_test_ggv_new/Controller/TrqVec_FLC_V2/Susp ==
  aSteerWheel : Inport
  vx : Inport  Port=2
  1-D Lookup Table : Lookup_n-D  NumberOfTableDimensions=1  BreakpointsForDimension1=Steer.Gain.vVehicle.Value  Table=Steer.Gain.n.Value  InterpMethod=Linear Lagrange  InternalRulePriority=Speed  RndMeth=Simplest
  Bus Creator{1..4} (4 alike) : BusCreator  Inputs=1
  Gain : Gain  Gain=3.6
  Product : Product
  Saturation : Saturate  UpperLimit=Steer.Limits.aUpper.Value  LowerLimit=Steer.Limits.aLower.Value  LinearizeAsGain=off  ZeroCross=off
  Transfer Fcn (with initial states) : simulink_extras/Additional Linear/Transfer Fcn (with initial states)  N=[1]  D="[1/Steer.fActuatorCutoff.Value  1]"  X0=-1
  SuspA1 : Outport  VectorParamsAs1DForOutWhenUnconnected=off
  SuspA2 : Outport  Port=2  VectorParamsAs1DForOutWhenUnconnected=off
  wires:
  1-D Lookup Table/1 -> Transfer Fcn (with initial states)/1
  Gain/1 -> 1-D Lookup Table/1
  Product/1 -> Saturation/1
  Transfer Fcn (with initial states)/1 -> Product/2
  vx/1 -> Gain/1
  Saturation/1 -> Bus Creator2/1  "aSteerWheel"
  aSteerWheel/1 -> Bus Creator4/1, Product/1  "aSteerWheel"
  Bus Creator1/1 -> SuspA1/1  "SuspA1"
  Bus Creator3/1 -> SuspA2/1  "SuspA2"
  Bus Creator2/1 -> Bus Creator3/1  "Steer"
  Bus Creator4/1 -> Bus Creator1/1  "Steer"

== system sm_car_test_ggv_new/Controller/TrqVec_FLC_V3/Brake Control ==
  "rBrakePedal " : Inport
  "VehBus " : Inport  Port=2
  Pedal : Subsystem  VariantControl=Pedal
  " Brakes" : Outport  VectorParamsAs1DForOutWhenUnconnected=off

== system sm_car_test_ggv_new/Controller/TrqVec_FLC_V3/Driveline Control ==
  Bus Creator : BusCreator  Inputs=1
  Constant : Constant  Value=0
  Driveline : Outport  VectorParamsAs1DForOutWhenUnconnected=off
  wires:
  Bus Creator/1 -> Driveline/1  "Driveline"
  Constant/1 -> Bus Creator/1  "placeholder"

== system sm_car_test_ggv_new/Controller/TrqVec_FLC_V3/Power Control ==
  rAccelPedal : Inport
  VehBus : Inport  Port=2
  aSteerWheel : Inport  Port=3
  Bus Creator : BusCreator  Inputs=2
  Bus Selector : BusSelector  OutputSignals=Chassis.SuspA2.LinkageL.Upright.Upright.w,Chassis.SuspA2.LinkageR.Upright.Upright.w
  Bus Selector1 : BusSelector  OutputSignals=v_x,a_x,a_y,phi_dot,v_y
  Data Type Conversion{,1..8} (9 alike) : DataTypeConversion  OutDataTypeStr=single  SaturateOnIntegerOverflow=off  RndMeth=Floor
  Data Type Conversion10 : DataTypeConversion  OutDataTypeStr=double  SaturateOnIntegerOverflow=off  RndMeth=Floor
  Data Type Conversion11 : DataTypeConversion  OutDataTypeStr=double  SaturateOnIntegerOverflow=off  RndMeth=Floor
  Gain : Gain  Gain=max(Control.MotorTrq)
  Gain1 : Gain  Gain=max(Control.MotorTrq)
  TV FLC V3 : Subsystem  TreatAsAtomicUnit=on  ReferencedSubsystem=TV_FLC_V3  MotorT=Control.MotorTrq  Gr=Control.GearRatio  MotorW=Control.MotorW  rwheel=Control.WheelRad  tr=Control.RearTrack  a=Control.FrontTrackToCG  a_cop=Control.FrontTrackToCoP  Af=Control.FrontalArea  cd=Control.LiftCoef  g=Control.GravitationalAcc  ro=Control.AirDensity  m=Control.Mass  h_CG=Control.CGHeight  L=Control.Wheelbase  Gain=Control.StrWheelRatio  Ku=Control.UndersteerGradient  F=Control.F  Slip_Ctrl_Kp=Control.Proportional_P  Slip_Ctrl_Ki=Control.Integral_I  Slip_Ctrl_Kd=Control.Derivative_D  Slip_Ctrl_Kn=Control.Filter_N  Load_Ref=Control.LoadRef  Slip_Ref=Control.SlipRef  FIS=Control.FuzzySystem  vx_th=Control.ActivationVelocity  Tmax=max(Control.MotorTrq)  C_alpha_F=Control.CalphaF  Slip_Steer_th=10  Kp_TV_Yaw=Control.Kp_Yaw  Kp_TV_Beta=Control.Kp_beta
  UKF State Estimation : Subsystem
  Power : Outport  VectorParamsAs1DForOutWhenUnconnected=off
  Out Bus Element : Outport  Port=2  PortName=Meas  Element=DYC
  Out Bus Element1 : Outport  Port=2  PortName=Meas  Element=UKF
  wires:
  VehBus/1 -> Bus Selector/1, UKF State Estimation/2(VehBus)
  Bus Selector/1 -> Data Type Conversion5/1  "<w>"
  Bus Selector/2 -> Data Type Conversion6/1  "<w>"
  rAccelPedal/1 -> Data Type Conversion8/1  "Throttle[~]"
  Bus Creator/1 -> Power/1
  TV FLC V3/1 -> Data Type Conversion10/1
  Gain/1 -> Bus Creator/1  "MMotorL2Demand"
  Gain1/1 -> Bus Creator/2  "MMotorR2Demand"
  aSteerWheel/1 -> Data Type Conversion/1, UKF State Estimation/1(aSteerWheel)
  TV FLC V3/2 -> Data Type Conversion11/1
  Data Type Conversion/1 -> TV FLC V3/1
  Data Type Conversion1/1 -> TV FLC V3/2
  Data Type Conversion2/1 -> TV FLC V3/3
  Data Type Conversion3/1 -> TV FLC V3/4
  Data Type Conversion4/1 -> TV FLC V3/5
  Data Type Conversion5/1 -> TV FLC V3/7
  Data Type Conversion6/1 -> TV FLC V3/8
  Data Type Conversion7/1 -> TV FLC V3/6
  Data Type Conversion8/1 -> TV FLC V3/9
  Data Type Conversion10/1 -> Gain/1
  Data Type Conversion11/1 -> Gain1/1
  TV FLC V3/3 -> Out Bus Element/1
  UKF State Estimation/1(StateEst) -> Bus Selector1/1
  Bus Selector1/1 -> Data Type Conversion1/1  "<v_x>"
  Bus Selector1/4 -> Data Type Conversion4/1  "<phi_dot>"
  Bus Selector1/2 -> Data Type Conversion2/1  "<a_x>"
  Bus Selector1/3 -> Data Type Conversion3/1  "<a_y>"
  Bus Selector1/5 -> Data Type Conversion7/1  "<v_y>"
  UKF State Estimation/2(Meas) -> Out Bus Element1/1  "Estimation"

== system sm_car_test_ggv_new/Controller/TrqVec_FLC_V3/Spring Damper ==
  Bus Creator : BusCreator  Inputs=4
  Bus Creator1 : BusCreator  Inputs=4
  Constant : Constant  Value=[0 0 0 0]
  Constant1 : Constant  Value=[0 0 0 0]
  Demux : Demux
  Demux1 : Demux
  Damper : Outport  VectorParamsAs1DForOutWhenUnconnected=off
  Spring : Outport  Port=2  VectorParamsAs1DForOutWhenUnconnected=off
  wires:
  Constant/1 -> Demux/1
  Demux/3 -> Bus Creator/3  "L2"
  Demux/4 -> Bus Creator/4  "R2"
  Demux/1 -> Bus Creator/1  "L1"
  Demux/2 -> Bus Creator/2  "R1"
  Demux1/2 -> Bus Creator1/2  "R1"
  Demux1/1 -> Bus Creator1/1  "L1"
  Demux1/4 -> Bus Creator1/4  "R2"
  Demux1/3 -> Bus Creator1/3  "L2"
  Constant1/1 -> Demux1/1
  Bus Creator1/1 -> Damper/1  "Damper"
  Bus Creator/1 -> Spring/1  "Spring"

== system sm_car_test_ggv_new/Controller/TrqVec_FLC_V3/Susp ==
  aSteerWheel : Inport
  vx : Inport  Port=2
  1-D Lookup Table : Lookup_n-D  NumberOfTableDimensions=1  BreakpointsForDimension1=Steer.Gain.vVehicle.Value  Table=Steer.Gain.n.Value  InterpMethod=Linear Lagrange  InternalRulePriority=Speed  RndMeth=Simplest
  Bus Creator{1..4} (4 alike) : BusCreator  Inputs=1
  Gain : Gain  Gain=3.6
  Product : Product
  Saturation : Saturate  UpperLimit=Steer.Limits.aUpper.Value  LowerLimit=Steer.Limits.aLower.Value  LinearizeAsGain=off  ZeroCross=off
  Transfer Fcn (with initial states) : simulink_extras/Additional Linear/Transfer Fcn (with initial states)  N=[1]  D="[1/Steer.fActuatorCutoff.Value  1]"  X0=-1
  SuspA1 : Outport  VectorParamsAs1DForOutWhenUnconnected=off
  SuspA2 : Outport  Port=2  VectorParamsAs1DForOutWhenUnconnected=off
  wires:
  Bus Creator4/1 -> Bus Creator1/1  "Steer"
  Bus Creator2/1 -> Bus Creator3/1  "Steer"
  Bus Creator3/1 -> SuspA2/1  "SuspA2"
  Bus Creator1/1 -> SuspA1/1  "SuspA1"
  aSteerWheel/1 -> Product/1, Bus Creator4/1  "aSteerWheel"
  Saturation/1 -> Bus Creator2/1  "aSteerWheel"
  vx/1 -> Gain/1
  Transfer Fcn (with initial states)/1 -> Product/2
  Product/1 -> Saturation/1
  Gain/1 -> 1-D Lookup Table/1
  1-D Lookup Table/1 -> Transfer Fcn (with initial states)/1
